simulink model "referenceFilter"  (R2020a)
settings: Solver=FixedStepAuto  StartTime=0.0  StopTime=10.0  FixedStep=0.2  RelTol=1e-3
settings Model: Creator=Admin  LastModifiedBy=Admin
settings DataIOCC: SaveOutput=off  SaveTime=off

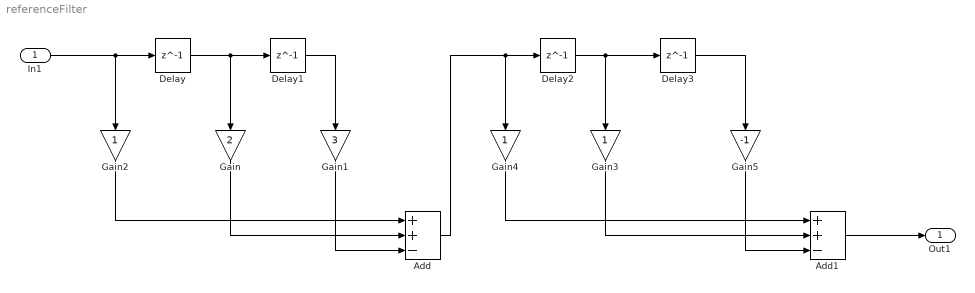
== system referenceFilter ==
  In1 : Inport  OutDataTypeStr=double  PortDimensions=1  SampleTime=[0.20000000000000001,0]
  Add : Sum  Inputs=++-
  Add1 : Sum  Inputs=++-
  Delay{,1..3} (4 alike) : Delay  DelayLength=1
  Gain : Gain  Gain=2
  Gain1 : Gain  Gain=3
  Gain2 : Gain
  Gain3 : Gain
  Gain4 : Gain
  Gain5 : Gain  Gain=-1
  Out1 : Outport  OutDataTypeStr=double  PortDimensions=1  SampleTime=[0.20000000000000001,0]
  wires:
  Delay2/1 -> Delay3/1, Gain3/1
  Add/1 -> Delay2/1, Gain4/1
  Gain2/1 -> Add/1
  Delay/1 -> Delay1/1, Gain/1
  Delay1/1 -> Gain1/1
  Gain1/1 -> Add/3
  Gain3/1 -> Add1/2
  Gain/1 -> Add/2
  Delay3/1 -> Gain5/1
  In1/1 -> Delay/1, Gain2/1
  Gain4/1 -> Add1/1
  Gain5/1 -> Add1/3
  Add1/1 -> Out1/1
